simulink model "Experiment"  (R2015a)
settings: Solver=ode1  StartTime=0.0  StopTime=inf  FixedStep=0.001  RelTol=1e-3
values from neighbouring files (symbols this model uses):
  ALPHA_MAX = 5.0 * pi/180    (= 0.0872664625997)    [Setup_exp.m]
  K_AMP = 1    [Setup_exp.m]    (also in Setup_sim.m)
  K_CT = lqr(Ai,Bi,Qx,Qu)    [Setup_sim.m]
  K_ENC_2DIP = [-1,1].*K_ENC_2DP    [Setup_exp.m]
  qc_get_step_size = 0.001    [Setup_exp.m]
  sysc = ss(A,B,C,D)    [Setup_sim.m]
  THETA_MAX = 35 * pi/180    (= 0.610865238198)    [Setup_exp.m]
  VMAX_DAC = 10    [Setup_exp.m]    (also in Setup_sim.m)
undefined symbols (not defined in the file or in its folder): HIL, K_ENC, L_CT, VMAX_AMP
libraries: simulink_extras x12, quarc_library x9, simulink x1
settings Model: SimulationMode=external  ExtModeTrigDuration=5000  Creator=MLevis  LastModifiedBy=labb2
settings SolverCC: PositivePriorityOrder=on
settings DataIOCC: SignalLoggingSaveFormat=ModelDataLogs
settings OptimizationCC: BooleanDataType=off  OptimizeBlockIOStorage=off  BufferReuse=off  GlobalBufferReuse=off  ExpressionFolding=off  ExpressionDepthLimit=2147483647  LocalBlockOutputs=off  InitFltsAndDblsToZero=on
settings DebuggingCC: SaveWithParameterizedLinksMsg=none  UnderspecifiedInitializationDetection=Classic  MergeDetectMultiDrivingBlocksExec=none  SignalResolutionControl=TryResolveAllWithWarning  MultiTaskDSMMsg=warning  MultiTaskCondExecSysMsg=none  FcnCallInpInsideContextMsg=UseLocalSettings  StateNameClashWarn=warning
settings HardwareCC: TargetHWDeviceType=32-bit Generic
settings RTWCC: SystemTargetFile=quarc_win64.tlc  TemplateMakefile=quarc_default_tmf  Description=QUARC Win64 Target
settings STFCustomTargetCC: TargetLibSuffix=.lib  TargetPreCompLibLocation=C:\PROGRA~3\QUARC\lib\2015a\win64\release  GenerateSampleERTMain=off  ConcurrentExecutionCompliant=on  GeneratePreprocessorConditionals=Disable all  ERTCustomFileBanners=off  SupportNonInlinedSFcns=on  SupportVariableSizeSignals=off  MATLABClassNameForMDSCustomization=Simulink.SoftwareTarget.GRTCustomization  CPPClassGenCompliant=on  GRTInterface=on  SystemTargetFile=quarc_win64.tlc
settings GRTTargetCC: TargetPreCompLibLocation=C:\PROGRA~3\QUARC\lib\2015a\win64\release  ParMdlRefBuildCompliant=off  CompOptLevelCompliant=off  CombineOutputUpdateFcns=off  MatFileLogging=off  GRTInterface=on  ExtMode=on  ExtModeMexFile=quarc_comm

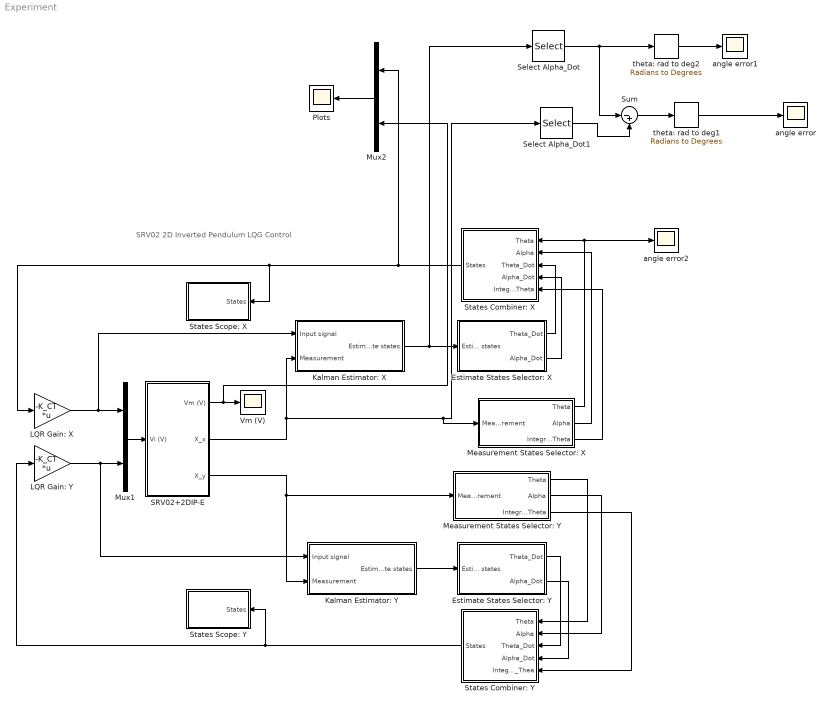
== system Experiment ==
  note: SRV02 2D Inverted Pendulum LQG Control
  Estimate States Selector: X : Subsystem
  Estimate States Selector: Y : Subsystem
  Kalman Estimator: X : Subsystem
  Kalman Estimator: Y : Subsystem
  LQR Gain: X : Gain  Gain=-K_CT  Multiplication=Matrix(K*u)  SaturateOnIntegerOverflow=on  OutDataTypeStr=Inherit: Same as input  ParamDataTypeStr=Inherit: Same as input
  LQR Gain: Y : Gain  Gain=-K_CT  Multiplication=Matrix(K*u)  SaturateOnIntegerOverflow=on  OutDataTypeStr=Inherit: Same as input  ParamDataTypeStr=Inherit: Same as input
  Measurement States Selector: X : Subsystem
  Measurement States Selector: Y : Subsystem
  Mux1 : Mux  Inputs=2
  Mux2 : Mux  Inputs=2
  Plots : Scope
      settings: TimeRange=60  YMin=-7.5  YMax=2  SaveName=data_theta5
  SRV02+2DIP-E : Subsystem
  Select Alpha_Dot : Selector  InputPortWidth=4  Indices=[1 2]
  Select Alpha_Dot1 : Selector  InputPortWidth=3  Indices=[1 2]
  States Combiner: X : Subsystem
  States Combiner: Y : Subsystem
  States Scope: X : Subsystem
  States Scope: Y : Subsystem
  Sum : Sum  Inputs=|-+
  Vm (V) : Scope
      settings: TickLabels=on  TimeRange=20  YMin=-0.7  YMax=1.4  SaveName=data_vm2
  angle error : Scope
      settings: TickLabels=on  TimeRange=20  YMin=-1.75  YMax=0.75  SaveName=data_vm
  angle error1 : Scope
      settings: TickLabels=on  TimeRange=20  YMin=-15  YMax=12.5  SaveName=data_vm1
  angle error2 : Scope
      settings: TickLabels=on  TimeRange=20  YMin=-1.75  YMax=0.75  SaveName=data_vm3
  theta: rad to deg1 : simulink_extras/Transformations/Radians to Degrees
  theta: rad to deg2 : simulink_extras/Transformations/Radians to Degrees
  wires:
  SRV02+2DIP-E/1(Vm (V)) -> Mux2/2, Vm (V)/1
  LQR Gain: X/1 -> Mux1/1, Kalman Estimator: X/1(Input signal)
  LQR Gain: Y/1 -> Kalman Estimator: Y/1(Input signal), Mux1/2
  Mux1/1 -> SRV02+2DIP-E/1(Vi (V))
  States Combiner: X/1(States) -> Mux2/1, LQR Gain: X/1, States Scope: X/1(States)
  Measurement States Selector: X/1(Theta) -> States Combiner: X/1(Theta), angle error2/1
  Measurement States Selector: X/2(Alpha) -> States Combiner: X/2(Alpha)
  Measurement States Selector: X/3(Integral_Theta) -> States Combiner: X/5(Integral_Theta)
  SRV02+2DIP-E/3(X_y) -> Kalman Estimator: Y/2(Measurement), Measurement States Selector: Y/1(Measurement)
  Kalman Estimator: Y/1(Estimate states) -> Estimate States Selector: Y/1(Estimate states)
  Measurement States Selector: Y/1(Theta) -> States Combiner: Y/1(Theta)
  Measurement States Selector: Y/2(Alpha) -> States Combiner: Y/2(Alpha)
  Measurement States Selector: Y/3(Integral_Theta) -> States Combiner: Y/5(Integral_Thea)
  States Combiner: Y/1(States) -> LQR Gain: Y/1, States Scope: Y/1(States)
  Estimate States Selector: Y/1(Theta_Dot) -> States Combiner: Y/3(Theta_Dot)
  Estimate States Selector: Y/2(Alpha_Dot) -> States Combiner: Y/4(Alpha_Dot)
  Estimate States Selector: X/1(Theta_Dot) -> States Combiner: X/3(Theta_Dot)
  Estimate States Selector: X/2(Alpha_Dot) -> States Combiner: X/4(Alpha_Dot)
  SRV02+2DIP-E/2(X_x) -> Kalman Estimator: X/2(Measurement), Select Alpha_Dot1/1, Measurement States Selector: X/1(Measurement)
  Kalman Estimator: X/1(Estimate states) -> Select Alpha_Dot/1, Estimate States Selector: X/1(Estimate states)
  Mux2/1 -> Plots/1
  Select Alpha_Dot/1 -> theta: rad to deg2/1, Sum/1
  Select Alpha_Dot1/1 -> Sum/2
  Sum/1 -> theta: rad to deg1/1
  theta: rad to deg1/1 -> angle error/1
  theta: rad to deg2/1 -> angle error1/1

== system Experiment/Estimate States Selector: X ==
  Estimate states : Inport
  Select Alpha_Dot : Selector  InputPortWidth=4  Indices=4
  Select Theta_Dot : Selector  InputPortWidth=4  Indices=3
  Theta_Dot : Outport
  Alpha_Dot : Outport  Port=2
  wires:
  Select Theta_Dot/1 -> Theta_Dot/1
  Select Alpha_Dot/1 -> Alpha_Dot/1
  Estimate states/1 -> Select Theta_Dot/1, Select Alpha_Dot/1

== system Experiment/Estimate States Selector: Y ==
  Estimate states : Inport
  Select Alpha_Dot : Selector  InputPortWidth=4  Indices=4
  Select Theta_Dot : Selector  InputPortWidth=4  Indices=3
  Theta_Dot : Outport
  Alpha_Dot : Outport  Port=2
  wires:
  Estimate states/1 -> Select Alpha_Dot/1, Select Theta_Dot/1
  Select Alpha_Dot/1 -> Alpha_Dot/1
  Select Theta_Dot/1 -> Theta_Dot/1

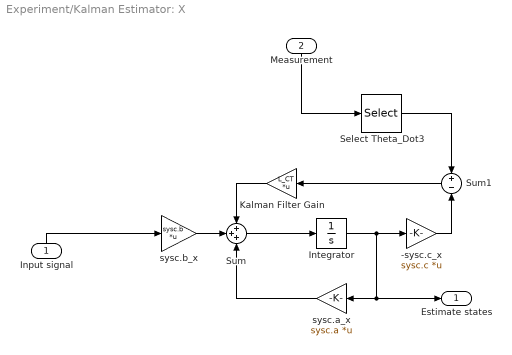
== system Experiment/Kalman Estimator: X ==
  Input signal : Inport
  Measurement : Inport  Port=2
  -sysc.c_x : Gain  Gain=sysc.c  Multiplication=Matrix(K*u)
  Integrator : Integrator
  Kalman Filter Gain : Gain  Gain=L_CT  Multiplication=Matrix(K*u)
  Select Theta_Dot3 : Selector  InputPortWidth=3  Indices=[1 2]
  Sum : Sum  Inputs=+++
  Sum1 : Sum  Inputs=+|-
  sysc.a_x : Gain  Gain=sysc.a  Multiplication=Matrix(K*u)
  sysc.b_x : Gain  Gain=sysc.b  Multiplication=Matrix(K*u)
  Estimate states : Outport
  wires:
  sysc.b_x/1 -> Sum/2
  Integrator/1 -> Estimate states/1, sysc.a_x/1, -sysc.c_x/1
  Sum/1 -> Integrator/1
  Kalman Filter Gain/1 -> Sum/1
  sysc.a_x/1 -> Sum/3
  Sum1/1 -> Kalman Filter Gain/1
  -sysc.c_x/1 -> Sum1/2
  Measurement/1 -> Select Theta_Dot3/1
  Input signal/1 -> sysc.b_x/1
  Select Theta_Dot3/1 -> Sum1/1

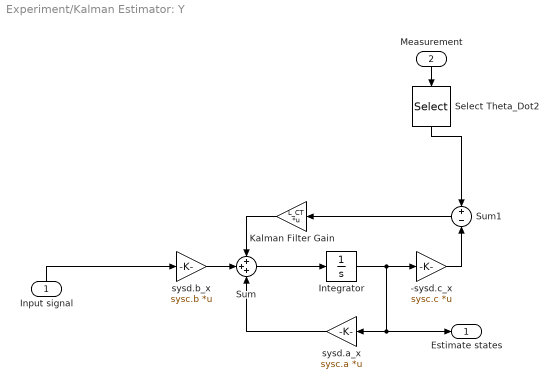
== system Experiment/Kalman Estimator: Y ==
  Input signal : Inport
  Measurement : Inport  Port=2
  -sysd.c_x : Gain  Gain=sysc.c  Multiplication=Matrix(K*u)
  Integrator : Integrator
  Kalman Filter Gain : Gain  Gain=L_CT  Multiplication=Matrix(K*u)
  Select Theta_Dot2 : Selector  InputPortWidth=3  Indices=[1 2]
  Sum : Sum  Inputs=+++
  Sum1 : Sum  Inputs=+|-
  sysd.a_x : Gain  Gain=sysc.a  Multiplication=Matrix(K*u)
  sysd.b_x : Gain  Gain=sysc.b  Multiplication=Matrix(K*u)
  Estimate states : Outport
  wires:
  Measurement/1 -> Select Theta_Dot2/1
  -sysd.c_x/1 -> Sum1/2
  Sum1/1 -> Kalman Filter Gain/1
  sysd.a_x/1 -> Sum/3
  Kalman Filter Gain/1 -> Sum/1
  Sum/1 -> Integrator/1
  Integrator/1 -> -sysd.c_x/1, sysd.a_x/1, Estimate states/1
  sysd.b_x/1 -> Sum/2
  Input signal/1 -> sysd.b_x/1
  Select Theta_Dot2/1 -> Sum1/1

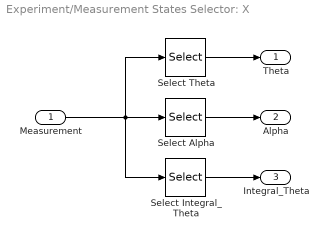
== system Experiment/Measurement States Selector: X ==
  Measurement : Inport
  Select Alpha : Selector  InputPortWidth=3  Indices=2
  Select Integral_Theta : Selector  InputPortWidth=3  Indices=3
  Select Theta : Selector  InputPortWidth=3
  Theta : Outport
  Alpha : Outport  Port=2
  Integral_Theta : Outport  Port=3
  wires:
  Select Theta/1 -> Theta/1
  Select Alpha/1 -> Alpha/1
  Select Integral_Theta/1 -> Integral_Theta/1
  Measurement/1 -> Select Alpha/1, Select Integral_Theta/1, Select Theta/1

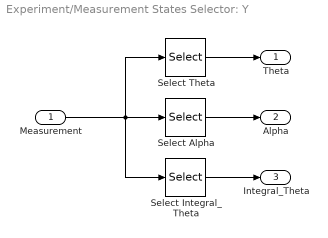
== system Experiment/Measurement States Selector: Y ==
  Measurement : Inport
  Select Alpha : Selector  InputPortWidth=3  Indices=2
  Select Integral_Theta : Selector  InputPortWidth=3  Indices=3
  Select Theta : Selector  InputPortWidth=3
  Theta : Outport
  Alpha : Outport  Port=2
  Integral_Theta : Outport  Port=3
  wires:
  Measurement/1 -> Select Theta/1, Select Integral_Theta/1, Select Alpha/1
  Select Integral_Theta/1 -> Integral_Theta/1
  Select Alpha/1 -> Alpha/1
  Select Theta/1 -> Theta/1

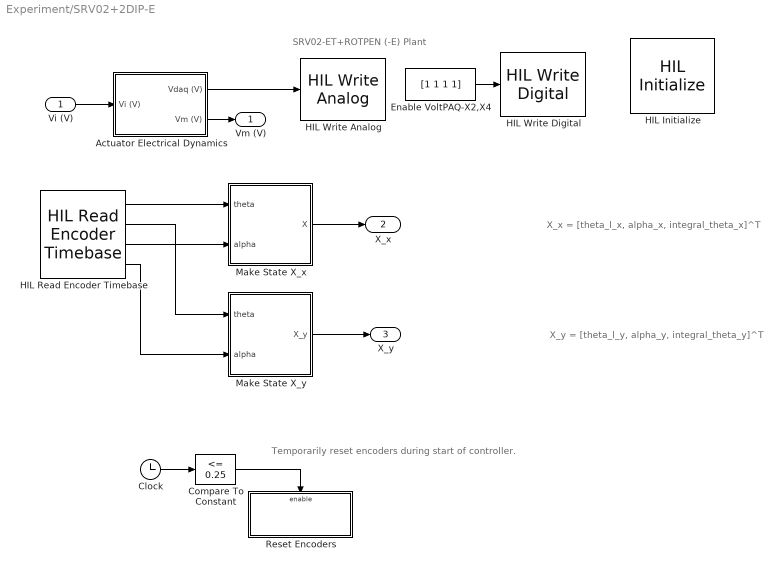
== system Experiment/SRV02+2DIP-E ==
  note: X_x = [theta_l_x, alpha_x, integral_theta_x]^T
  note: SRV02-ET+ROTPEN (-E) Plant
  note: X_y = [theta_l_y, alpha_y, integral_theta_y]^T
  note: Temporarily reset encoders during start of controller.
  Vi (V) : Inport
  Actuator Electrical Dynamics : Subsystem
  Clock : Clock
  Compare To Constant : simulink/Logic and Bit Operations/Compare To Constant  relop=<=  const=0.25  OutDataTypeStr=uint8  ZeroCross=off
  Enable VoltPAQ-X2,X4 : Constant  Value=[1 1 1 1]
  HIL Initialize : quarc_library/Data Acquisition/Generic/Configuration/HIL Initialize  object_name=HIL-1  board_type=q8_usb  board_number=0  board_options=update_rate=normal  exclusive=off  active=off  hardware_clocks=[0:2]  clock_modes=[]  initial_clock_frequencies=[]  set_clock_params_at_start=off  set_clock_params_at_switch_in=off  set_clock_frequencies_at_start=off  set_clock_frequencies_at_switch_in=off  analog_input_channels=[0:7]  analog_input_maximums=10  analog_input_minimums=-10  set_analog_input_params_at_start=on  set_analog_input_params_at_switch_in=off  analog_output_channels=[0:7]  analog_output_maximums=10  analog_output_minimums=-10  initial_analog_outputs=[0]  final_analog_outputs=[0]  watchdog_analog_outputs=0  set_analog_output_params_at_start=on  set_analog_output_params_at_switch_in=off  set_analog_outputs_at_start=on  set_analog_outputs_at_switch_in=off  set_analog_outputs_at_terminate=on  set_analog_outputs_at_switch_out=off  set_analog_outputs_on_watchdog=off  digital_input_channels=[]  digital_output_channels=[0:7]  digital_output_configuration=[]  initial_digital_outputs=[0]  final_digital_outputs=[0]  watchdog_digital_outputs=[0]  set_digital_output_params_at_start=off  set_digital_output_params_at_switch_in=off  set_digital_outputs_at_start=on  set_digital_outputs_at_switch_in=off  set_digital_outputs_at_terminate=on  set_digital_outputs_at_switch_out=off  set_digital_outputs_on_watchdog=off  encoder_channels=[0:7]  quadrature=[4]  encoder_filter_frequency=[]  initial_encoder_counts=[0]  set_encoder_params_at_start=on  set_encoder_params_at_switch_in=off  set_encoder_counts_at_start=on  set_encoder_counts_at_switch_in=off  pwm_channels=[0:7]  pwm_modes=0  pwm_frequency=99.532799999999995e6/4095  pwm_configuration=[0]  pwm_alignment=[0]  pwm_polarity=[1]  pwm_leading_deadband=[0]  pwm_trailing_deadband=[0]  initial_pwm_outputs=[0]  final_pwm_outputs=[0]  watchdog_pwm_outputs=[0]  set_pwm_params_at_start=on  set_pwm_params_at_switch_in=off  set_pwm_outputs_at_start=on  set_pwm_outputs_at_switch_in=off  set_pwm_outputs_at_terminate=on  set_pwm_outputs_at_switch_out=off  set_pwm_outputs_on_watchdog=off  other_output_channels=[]  initial_other_outputs=[]  final_other_outputs=[]  watchdog_other_outputs=[]  set_other_outputs_at_start=off  set_other_outputs_at_switch_in=off  set_other_outputs_at_terminate=off  set_other_outputs_at_switch_out=off  set_other_outputs_on_watchdog=off
  HIL Read Encoder Timebase : quarc_library/Data Acquisition/Generic/Timebases/HIL Read Encoder Timebase  object_name=HIL-1  clock=0  channels=0:3  samples_in_buffer=max(ceil(1/qc_get_step_size), 1)  active=on  vector_output=off  data_type_mode=Inherit via back propagation  data_type=double
  HIL Write Analog : quarc_library/Data Acquisition/Generic/Immediate I//O/HIL Write Analog  object_name=HIL-1  channels=[0,1]  sample_time=-1  active=off  vector_input=on
  HIL Write Digital : quarc_library/Data Acquisition/Generic/Immediate I//O/HIL Write Digital  object_name=HIL-1  channels=[0:3]  sample_time=-1  active=off  vector_input=on
  Make State X_x : Subsystem
  Make State X_y : Subsystem
  Reset Encoders : Subsystem  TreatAsAtomicUnit=on
  Vm (V) : Outport  InitialOutput=0
  X_x : Outport  Port=2  InitialOutput=0
  X_y : Outport  Port=3  InitialOutput=0
  wires:
  Make State X_x/1(X) -> X_x/1
  Vi (V)/1 -> Actuator Electrical Dynamics/1(Vi (V))
  Actuator Electrical Dynamics/1(Vdaq (V)) -> HIL Write Analog/1
  HIL Read Encoder Timebase/1 -> Make State X_x/1(theta)
  HIL Read Encoder Timebase/2 -> Make State X_y/1(theta)
  HIL Read Encoder Timebase/3 -> Make State X_x/2(alpha)
  HIL Read Encoder Timebase/4 -> Make State X_y/2(alpha)
  Make State X_y/1(X_y) -> X_y/1
  Clock/1 -> Compare To Constant/1
  Compare To Constant/1 -> Reset Encoders/Enable
  Actuator Electrical Dynamics/2(Vm (V)) -> Vm (V)/1
  Enable VoltPAQ-X2,X4/1 -> HIL Write Digital/1

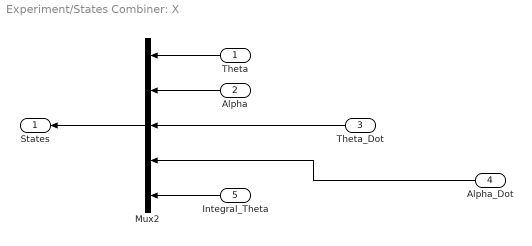
== system Experiment/States Combiner: X ==
  Theta : Inport
  Alpha : Inport  Port=2
  Theta_Dot : Inport  Port=3
  Alpha_Dot : Inport  Port=4
  Integral_Theta : Inport  Port=5
  Mux2 : Mux  Inputs=5
  States : Outport
  wires:
  Mux2/1 -> States/1
  Integral_Theta/1 -> Mux2/5
  Alpha/1 -> Mux2/2
  Theta/1 -> Mux2/1
  Theta_Dot/1 -> Mux2/3
  Alpha_Dot/1 -> Mux2/4

== system Experiment/States Combiner: Y ==
  Theta : Inport
  Alpha : Inport  Port=2
  Theta_Dot : Inport  Port=3
  Alpha_Dot : Inport  Port=4
  Integral_Thea : Inport  Port=5
  Mux2 : Mux  Inputs=5
  States : Outport
  wires:
  Theta/1 -> Mux2/1
  Alpha/1 -> Mux2/2
  Integral_Thea/1 -> Mux2/5
  Mux2/1 -> States/1
  Alpha_Dot/1 -> Mux2/4
  Theta_Dot/1 -> Mux2/3

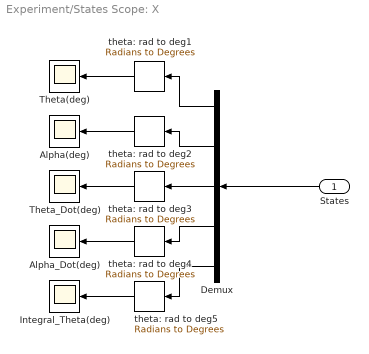
== system Experiment/States Scope: X ==
  States : Inport
  Alpha(deg) : Scope
      settings: TimeRange=300  YMin=-3.5  YMax=0.5  SaveName=data_theta1
  Alpha_Dot(deg) : Scope
      settings: TimeRange=300  YMin=-30  YMax=-16  SaveName=data_theta3
  Demux : Demux  Outputs=5
  Integral_Theta(deg) : Scope
      settings: TimeRange=300  YMin=-57.5  YMax=-49.5  SaveName=data_theta4
  Theta(deg) : Scope
      settings: TimeRange=300  YMin=-20  YMax=20  SaveName=data_theta
  Theta_Dot(deg) : Scope
      settings: TimeRange=300  YMin=-70  YMax=40  SaveName=data_theta2
  theta: rad to deg{1..5} (5 alike) : simulink_extras/Transformations/Radians to Degrees
  wires:
  States/1 -> Demux/1
  theta: rad to deg1/1 -> Theta(deg)/1
  Demux/1 -> theta: rad to deg1/1
  theta: rad to deg2/1 -> Alpha(deg)/1
  theta: rad to deg3/1 -> Theta_Dot(deg)/1
  theta: rad to deg4/1 -> Alpha_Dot(deg)/1
  theta: rad to deg5/1 -> Integral_Theta(deg)/1
  Demux/2 -> theta: rad to deg2/1
  Demux/3 -> theta: rad to deg3/1
  Demux/4 -> theta: rad to deg4/1
  Demux/5 -> theta: rad to deg5/1

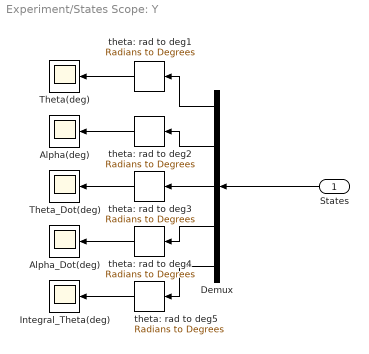
== system Experiment/States Scope: Y ==
  States : Inport
  Alpha(deg) : Scope
      settings: TimeRange=300  YMin=-17074.06908  YMax=153616.62176  SaveName=data_theta1
  Alpha_Dot(deg) : Scope
      settings: TimeRange=300  YMin=-17074.06908  YMax=153616.62176  SaveName=data_theta3
  Demux : Demux  Outputs=5
  Integral_Theta(deg) : Scope
      settings: TimeRange=300  YMin=-17074.06908  YMax=153616.62176  SaveName=data_theta4
  Theta(deg) : Scope
      settings: TimeRange=300  YMin=-17074.06908  YMax=153616.62176  SaveName=data_theta
  Theta_Dot(deg) : Scope
      settings: TimeRange=300  YMin=-17074.06908  YMax=153616.62176  SaveName=data_theta2
  theta: rad to deg{1..5} (5 alike) : simulink_extras/Transformations/Radians to Degrees
  wires:
  Demux/5 -> theta: rad to deg5/1
  Demux/4 -> theta: rad to deg4/1
  Demux/3 -> theta: rad to deg3/1
  Demux/2 -> theta: rad to deg2/1
  theta: rad to deg5/1 -> Integral_Theta(deg)/1
  theta: rad to deg4/1 -> Alpha_Dot(deg)/1
  theta: rad to deg3/1 -> Theta_Dot(deg)/1
  theta: rad to deg2/1 -> Alpha(deg)/1
  Demux/1 -> theta: rad to deg1/1
  theta: rad to deg1/1 -> Theta(deg)/1
  States/1 -> Demux/1

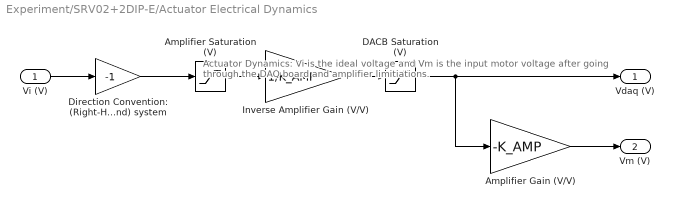
== system Experiment/SRV02+2DIP-E/Actuator Electrical Dynamics ==
  note: Actuator Dynamics: Vi is the ideal voltage and Vm is the
      | input motor voltage after going through the DAQ board and amplifier limitiations.
  Vi (V) : Inport
  Amplifier Gain (V/V) : Gain  Gain=-K_AMP
  Amplifier Saturation (V) : Saturate  UpperLimit=VMAX_AMP  LowerLimit=-VMAX_AMP
  DACB Saturation (V) : Saturate  UpperLimit=VMAX_DAC  LowerLimit=-VMAX_DAC
  Direction Convention: (Right-Hand) system : Gain  Gain=-1  SaturateOnIntegerOverflow=on  OutDataTypeStr=Inherit: Same as input  ParamDataTypeStr=Inherit: Same as input
  Inverse Amplifier Gain (V/V) : Gain  Gain=1/K_AMP
  Vdaq (V) : Outport
  Vm (V) : Outport  Port=2
  wires:
  Direction Convention: (Right-Hand) system/1 -> Amplifier Saturation (V)/1
  Amplifier Gain (V/V)/1 -> Vm (V)/1
  DACB Saturation (V)/1 -> Vdaq (V)/1, Amplifier Gain (V/V)/1
  Inverse Amplifier Gain (V/V)/1 -> DACB Saturation (V)/1
  Vi (V)/1 -> Direction Convention: (Right-Hand) system/1
  Amplifier Saturation (V)/1 -> Inverse Amplifier Gain (V/V)/1

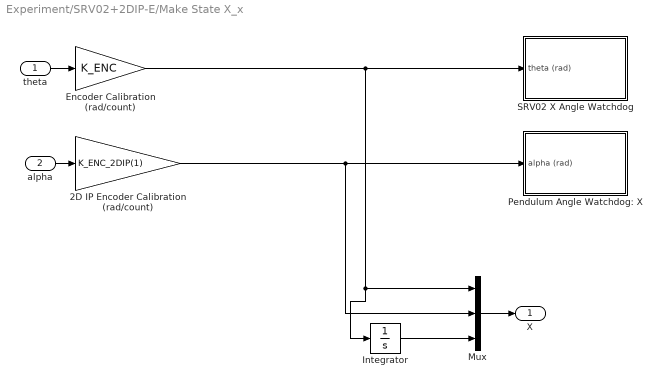
== system Experiment/SRV02+2DIP-E/Make State X_x ==
  theta : Inport
  alpha : Inport  Port=2
  2D IP Encoder Calibration (rad/count) : Gain  Gain=K_ENC_2DIP(1)  SaturateOnIntegerOverflow=on  OutDataTypeStr=Inherit: Same as input  ParamDataTypeStr=Inherit: Same as input
  Encoder Calibration (rad/count) : Gain  Gain=K_ENC  SaturateOnIntegerOverflow=on  OutDataTypeStr=Inherit: Same as input  ParamDataTypeStr=Inherit: Same as input
  Integrator : Integrator
  Mux : Mux  Inputs=3
  Pendulum Angle Watchdog: X : Subsystem  TreatAsAtomicUnit=on
  SRV02 X Angle Watchdog : Subsystem  TreatAsAtomicUnit=on
  X : Outport
  wires:
  alpha/1 -> 2D IP Encoder Calibration (rad/count)/1
  theta/1 -> Encoder Calibration (rad/count)/1
  2D IP Encoder Calibration (rad/count)/1 -> Pendulum Angle Watchdog: X/1(alpha (rad)), Mux/2
  Encoder Calibration (rad/count)/1 -> Integrator/1, Mux/1, SRV02 X Angle Watchdog/1(theta (rad))
  Mux/1 -> X/1
  Integrator/1 -> Mux/3

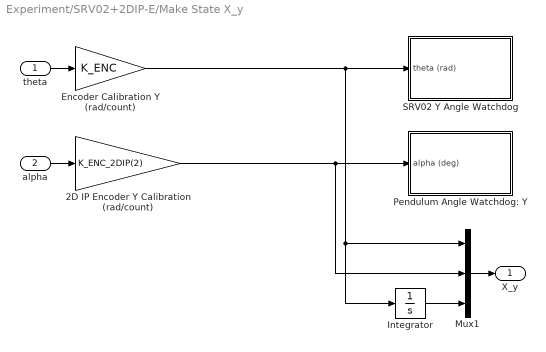
== system Experiment/SRV02+2DIP-E/Make State X_y ==
  theta : Inport
  alpha : Inport  Port=2
  2D IP Encoder Y Calibration (rad/count) : Gain  Gain=K_ENC_2DIP(2)  SaturateOnIntegerOverflow=on  OutDataTypeStr=Inherit: Same as input  ParamDataTypeStr=Inherit: Same as input
  Encoder Calibration Y (rad/count) : Gain  Gain=K_ENC  SaturateOnIntegerOverflow=on  OutDataTypeStr=Inherit: Same as input  ParamDataTypeStr=Inherit: Same as input
  Integrator : Integrator
  Mux1 : Mux  Inputs=3
  Pendulum Angle Watchdog: Y : Subsystem  TreatAsAtomicUnit=on
  SRV02 Y Angle Watchdog : Subsystem  TreatAsAtomicUnit=on
  X_y : Outport  InitialOutput=0
  wires:
  Encoder Calibration Y (rad/count)/1 -> Integrator/1, Mux1/1, SRV02 Y Angle Watchdog/1(theta (rad))
  2D IP Encoder Y Calibration (rad/count)/1 -> Pendulum Angle Watchdog: Y/1(alpha (deg)), Mux1/2
  alpha/1 -> 2D IP Encoder Y Calibration (rad/count)/1
  theta/1 -> Encoder Calibration Y (rad/count)/1
  Mux1/1 -> X_y/1
  Integrator/1 -> Mux1/3

== system Experiment/SRV02+2DIP-E/Reset Encoders ==
  Enable : EnablePort
  HIL Set Encoder Counts : quarc_library/Data Acquisition/Generic/Configuration/HIL Set Encoder Counts  object_name=HIL-1  channels=[0:3]  source=internal  counts=0  sample_time=qc_get_step_size  active=on  vector_input=off
      settings: AttributesFormatString=(%<object_name>)

== system Experiment/SRV02+2DIP-E/Make State X_x/Pendulum Angle Watchdog: X ==
  alpha (rad) : Inport
  Abs : Abs
  Check Maximum Allowed Angle : RelationalOperator  Operator=<  InputSameDT=on
  Stop with Message : quarc_library/Sinks/Error Handling/Stop with Message  message_type=Fixed error message  message_icon=Error  message=Maximum angle reached: pendulum x angle.
  X MAX : Constant  Value=ALPHA_MAX
  wires:
  Abs/1 -> Check Maximum Allowed Angle/2
  Check Maximum Allowed Angle/1 -> Stop with Message/1
  alpha (rad)/1 -> Abs/1
  X MAX/1 -> Check Maximum Allowed Angle/1

== system Experiment/SRV02+2DIP-E/Make State X_x/SRV02 X Angle Watchdog ==
  theta (rad) : Inport
  Abs : Abs
  Check Maximum Allowed Angle : RelationalOperator  Operator=<  InputSameDT=on
  Stop with Message : quarc_library/Sinks/Error Handling/Stop with Message  message_type=Fixed error message  message_icon=Error  message=Maximum angle reached: SRV02 X angle.
  X MAX : Constant  Value=THETA_MAX
  wires:
  X MAX/1 -> Check Maximum Allowed Angle/1
  theta (rad)/1 -> Abs/1
  Check Maximum Allowed Angle/1 -> Stop with Message/1
  Abs/1 -> Check Maximum Allowed Angle/2

== system Experiment/SRV02+2DIP-E/Make State X_y/Pendulum Angle Watchdog: Y ==
  alpha (deg) : Inport
  Abs : Abs
  Check Maximum Allowed Angle : RelationalOperator  Operator=<  InputSameDT=on
  Stop with Message : quarc_library/Sinks/Error Handling/Stop with Message  message_type=Fixed error message  message_icon=Error  message=Maximum angle reached: pendulum y angle.
  X MAX : Constant  Value=ALPHA_MAX
  wires:
  Abs/1 -> Check Maximum Allowed Angle/2
  Check Maximum Allowed Angle/1 -> Stop with Message/1
  alpha (deg)/1 -> Abs/1
  X MAX/1 -> Check Maximum Allowed Angle/1

== system Experiment/SRV02+2DIP-E/Make State X_y/SRV02 Y Angle Watchdog ==
  theta (rad) : Inport
  Abs : Abs
  Check Maximum Allowed Angle : RelationalOperator  Operator=<  InputSameDT=on
  Stop with Message : quarc_library/Sinks/Error Handling/Stop with Message  message_type=Fixed error message  message_icon=Error  message=Maximum angle reached: SRV02 Y angle.
  X MAX : Constant  Value=THETA_MAX
  wires:
  Abs/1 -> Check Maximum Allowed Angle/2
  Check Maximum Allowed Angle/1 -> Stop with Message/1
  theta (rad)/1 -> Abs/1
  X MAX/1 -> Check Maximum Allowed Angle/1
